simulink model "EnumAssignslx"  (R2021a)
settings: Solver=FixedStepDiscrete  StartTime=0.0  StopTime=10.0  RelTol=1e-3
settings Model: Creator=OmarMedhat  LastModifiedBy=OmarMedhat
settings OptimizationCC: DefaultParameterBehavior=Inlined  EnhancedBackFolding=on  PassReuseOutputArgsAs=Individual arguments  ZeroExternalMemoryAtStartup=off  ZeroInternalMemoryAtStartup=off  OptimizeBlockOrder=speed  DifferentSizesBufferReuse=on  OptimizationCustomize=off  EfficientTunableParamExpr=on
settings DebuggingCC: ParameterTunabilityLossMsg=error
settings SFSimCC: MATLABDynamicMemAlloc=off
settings RTWCC: SystemTargetFile=ert.tlc  GenCodeOnly=on  TemplateMakefile=ert_default_tmf  GenerateReport=on  IncludeHyperlinkInReport=on  LaunchReport=on  GenerateTraceInfo=on
settings CodeAppCC: ForceParamTrailComments=on  IgnoreCustomStorageClasses=off  OperatorAnnotations=on  SimulinkDataObjDesc=on  SFDataObjDesc=on  InsertBlockDesc=on
settings ERTTargetCC: TargetLangStandard=C99 (ISO)  GenerateSampleERTMain=on  InlinedParameterPlacement=NonHierarchical  ERTCustomFileTemplate=example_file_process.tlc

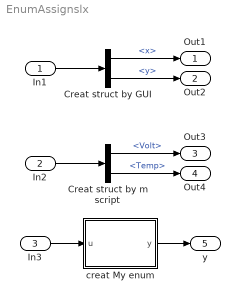
== system EnumAssignslx ==
  In1 : Inport  OutDataTypeStr=Bus: MYstr  BusOutputAsStruct=on
  In2 : Inport  Port=2  OutDataTypeStr=Bus: Fault  BusOutputAsStruct=on
  In3 : Inport  Port=3  OutDataTypeStr=Enum: enum1
  Creat struct by GUI : BusSelector  OutputSignals=x,y
  Creat struct by m script : BusSelector  OutputSignals=Volt,Temp
  creat My enum : MATLAB Function  TreatAsAtomicUnit=on
  Out1 : Outport
  Out2 : Outport  Port=2
  Out3 : Outport  Port=3
  Out4 : Outport  Port=4
  y : Outport  Port=5
  wires:
  In1/1 -> Creat struct by GUI/1
  Creat struct by GUI/1 -> Out1/1  "<x>"
  Creat struct by GUI/2 -> Out2/1  "<y>"
  Creat struct by m script/1 -> Out3/1  "<Volt>"
  Creat struct by m script/2 -> Out4/1  "<Temp>"
  In2/1 -> Creat struct by m script/1
  In3/1 -> creat My enum/1(u)
  creat My enum/1(y) -> y/1

== matlab function EnumAssignslx/creat My enum ==
  data: u input; y output
function y = fcn(u)

y = u;
